simulink model "item1"  (R2013a)
settings: Solver=ode45  StartTime=0.0  StopTime=1  RelTol=1e-3
undefined symbols (not defined in the file): B, J, Ke, Kt, La, Ra
settings Model: Creator=Guilherme  LastModifiedBy=Guilherme

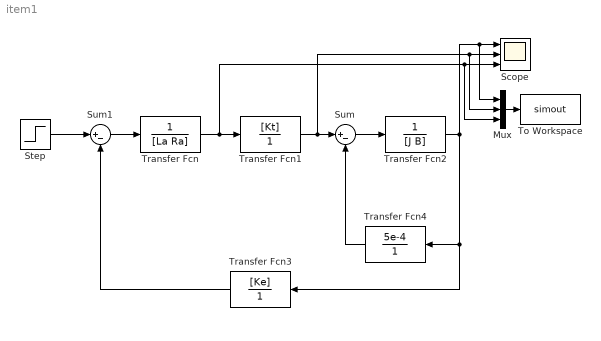
== system item1 ==
  Mux : Mux  Inputs=3
  Scope : Scope  NumInputPorts=3
      settings: YMin=-5~-5~-5  YMax=5~5~5
  Step : Step  Time=0.1  After=24  SampleTime=0
  Sum : Sum  Inputs=|+-
  Sum1 : Sum  Inputs=|+-
  To Workspace : ToWorkspace  VariableName=simout  SampleTime=-1  SaveFormat=Timeseries
  Transfer Fcn : TransferFcn  Denominator=[La Ra]
  Transfer Fcn1 : TransferFcn  Numerator=[Kt]  Denominator=[1]
  Transfer Fcn2 : TransferFcn  Denominator=[J B]
  Transfer Fcn3 : TransferFcn  Numerator=[Ke]  Denominator=[1]
  Transfer Fcn4 : TransferFcn  Numerator=[5e-4]  Denominator=[1]
  wires:
  Transfer Fcn/1 -> Mux/3, Scope/3, Transfer Fcn1/1
  Transfer Fcn1/1 -> Sum/1, Mux/2, Scope/2
  Sum/1 -> Transfer Fcn2/1
  Transfer Fcn2/1 -> Transfer Fcn3/1, Transfer Fcn4/1, Mux/1, Scope/1
  Transfer Fcn3/1 -> Sum1/2
  Sum1/1 -> Transfer Fcn/1
  Step/1 -> Sum1/1
  Mux/1 -> To Workspace/1
  Transfer Fcn4/1 -> Sum/2
